simulink model "CompletePhysicalTireSystem"  (R2025b)
settings: Solver=FixedStepAuto  StartTime=0.0  StopTime=150  FixedStep=0.001  RelTol=1e-3
undefined symbols (not defined in the file): const_mode, init_pressure
libraries: fl_lib x8, nesl_utility x7, SimscapeFluids_lib x3, simulink x1, slpidlib x1
(part 3 of 3)

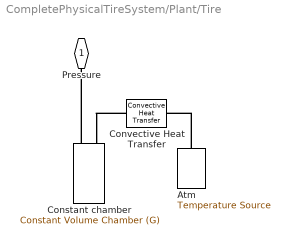
== system CompletePhysicalTireSystem/Plant/Tire ==
  Atm : fl_lib/Thermal/Thermal Sources/Temperature Source  temperature=293.15 K
  Constant chamber : fl_lib/Gas/Elements/Constant Volume Chamber (G)  volume=0.045 m^3  num_ports=foundation.enum.num_ports.one  area_A=0.01 m^2  area_B=0.01 m^2  area_C=0.01 m^2  area_D=0.01 m^2  p_I_specify=on  p_I_priority=High  p_I=init_pressure bar  p_I_nominal_specify=off  p_I_nominal_value=1  p_I_nominal_unit=MPa  T_I_specify=off  T_I_priority=High  T_I=293.15 K  T_I_nominal_specify=off  T_I_nominal_value=1  T_I_nominal_unit=K  rho_I_specify=off  rho_I_priority=None  rho_I=1.2 kg/m^3  rho_I_nominal_specify=off  rho_I_nominal_value=1  rho_I_nominal_unit=kg/m^3
      settings: InternalSimscapePortConfiguration="{\"Bottom\":[],\"Left\":[{\"id\":\"A\",\"label\":\"A\",\"type\":\"foundation.gas.gas\"},{\"id\":\"H\",\"label\":\"H\",\"type\":\"foundation.thermal.thermal\"}],\"Right\":[],\"Top\":[]}"
  Convective Heat Transfer : fl_lib/Thermal/Thermal Elements/Convective Heat Transfer  thermal_type=foundation.enum.constant_variable.constant  area=1e-4 m^2  heat_tr_coeff=20 W/(K*m^2)  min_heat_tr_coeff=1e-3 W/(K*m^2)  T_specify=off  T_priority=None  T=0 K  T_nominal_specify=off  T_nominal_value=1  T_nominal_unit=K  Q_specify=off  Q_priority=None  Q=0 W  Q_nominal_specify=off  Q_nominal_value=1  Q_nominal_unit=W
  Pressure : PMIOPort  Side=Left
  connections:
  Constant chamber/LConn1 -- Pressure/RConn1
  Convective Heat Transfer/LConn1 -- Constant chamber/LConn2
  Atm/LConn1 -- Convective Heat Transfer/RConn1

== stateflow chart CompletePhysicalTireSystem/Planner ==
  state Modes
    entry:
    Target_pressure = 2.7;
  state High_Speed
    entry:
    Target_pressure = 2.9;
  state High_friction
    entry:
    Target_pressure =2.5;
  (default) -> Modes
  Modes -> High_Speed [order 1] : [Mode == 1]
  Modes -> High_friction [order 2] : [Mode == 2]
  High_friction -> High_Speed : [Mode == 1]
  High_Speed -> High_friction : [Mode == 2]
  data: Target_pressure output; Mode input
